simulink model "SixCellImplementation"  (R2021b)
settings: Solver=VariableStepAuto  StartTime=0.0  StopTime=500  RelTol=1e-3
libraries: spsVoltageMeasurementLib x8, spsDiodeLib x6, spsSeriesRLCBranchLib x6, spsLinearTransformerLib x3, spsGroundLib x1, spsMosfetLib x1, spspowerguiLib x1
settings Model: Creator=HP  LastModifiedBy=rajra
settings SolverCC: ZeroCrossAlgorithm=Adaptive  AlgebraicLoopSolver=TrustRegion
settings DebuggingCC: IgnoredZcDiagnostic=none  SFMachineParentedDataDiag=warning

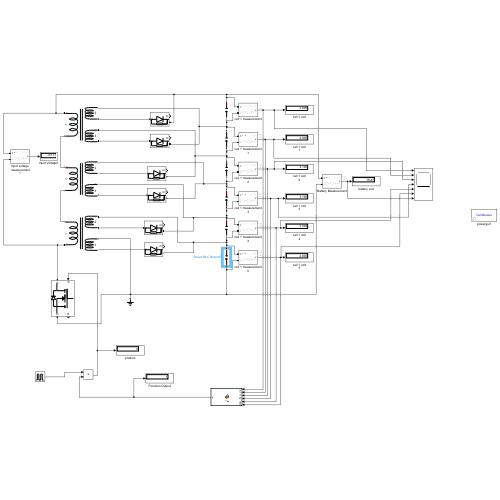
[thumbnail: Simulink's stored preview of the top-level diagram]
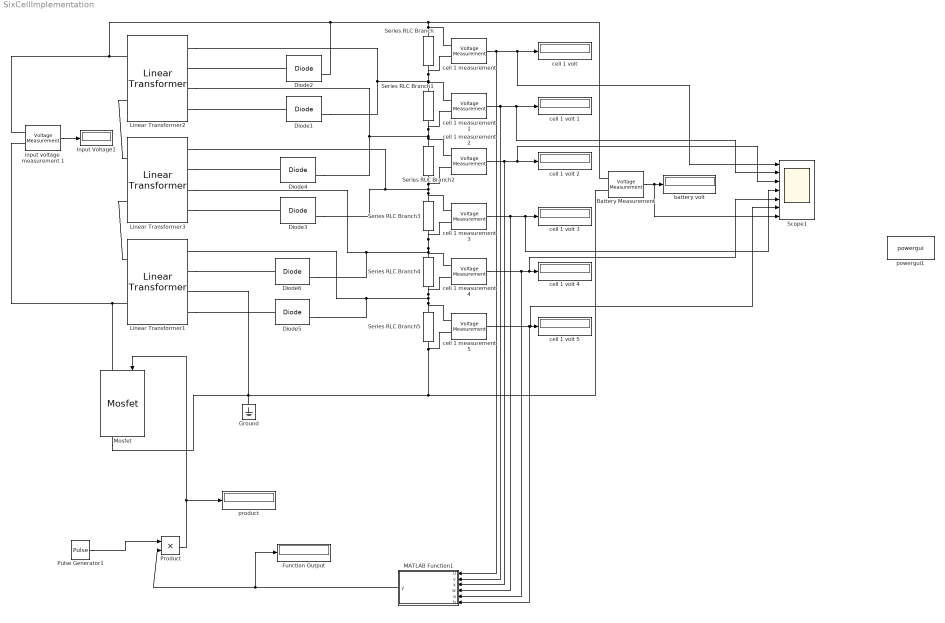
== system SixCellImplementation ==
  "Battery Measurement " : spsVoltageMeasurementLib/Voltage Measurement  PhasorSimulation=off  OutputType=Complex  PSBequivalent=0
  Diode{1..6} (6 alike) : spsDiodeLib/Diode  Ron=0.001  Lon=0  Vf=0.8  IC=0  UseSnubber=0  Rs=500  Cs=250e-9  Measurements=on
  Function Output : Display
  Ground : spsGroundLib/Ground  LConnTagsString=a
  Input Voltage1 : Display
  Linear Transformer1 : spsLinearTransformerLib/Linear Transformer  UNITS=SI  NominalPower=[100 55000]  winding1=[10 0.02 45e-6]  winding2=[5 0.02 288e-6]  ThreeWindings=on  winding3=[5 0.02 288e-6]  RmLm=[1.0805e+06 2866]  Measurements=None  DataType=on
  Linear Transformer2 : spsLinearTransformerLib/Linear Transformer  UNITS=SI  NominalPower=[100 55000]  winding1=[10 0.02 45e-6]  winding2=[5 0.02 288e-6]  ThreeWindings=on  winding3=[5 0.02 288e-6]  RmLm=[1.0805e+06 2866]  Measurements=None  DataType=on
  Linear Transformer3 : spsLinearTransformerLib/Linear Transformer  UNITS=SI  NominalPower=[100 55000]  winding1=[10 0.02 45e-6]  winding2=[5 0.02 288e-6]  ThreeWindings=on  winding3=[5 0.02 288e-6]  RmLm=[1.0805e+06 2866]  Measurements=None  DataType=on
  MATLAB Function1 : MATLAB Function  TreatAsAtomicUnit=on
  Mosfet : spsMosfetLib/Mosfet  Ron=1.5  Lon=0  Rd=2  Vfd=0  IC=0  Rs=1500  Cs=288e-7  Measurements=on
  Product : Product
  Pulse Generator1 : DiscretePulseGenerator  PulseType=Time based  Period=10  PulseWidth=50
  Scope1 : Scope  NumInputPorts=7
  Series RLC Branch : spsSeriesRLCBranchLib/Series RLC Branch  LConnTagsString=__new0  RConnTagsString=__new0  BranchType=C  Resistance=1  Inductance=1e-3  SetiL0=off  InitialCurrent=0  Capacitance=5  Setx0=on  InitialVoltage=3  Measurements=None
  Series RLC Branch1 : spsSeriesRLCBranchLib/Series RLC Branch  LConnTagsString=__new0  RConnTagsString=__new0  BranchType=C  Resistance=1  Inductance=1e-3  SetiL0=off  InitialCurrent=0  Capacitance=5  Setx0=on  InitialVoltage=3.0  Measurements=None
  Series RLC Branch2 : spsSeriesRLCBranchLib/Series RLC Branch  LConnTagsString=__new0  RConnTagsString=__new0  BranchType=C  Resistance=1  Inductance=1e-3  SetiL0=off  InitialCurrent=0  Capacitance=5  Setx0=on  InitialVoltage=3.2  Measurements=None
  Series RLC Branch3 : spsSeriesRLCBranchLib/Series RLC Branch  LConnTagsString=__new0  RConnTagsString=__new0  BranchType=C  Resistance=1  Inductance=1e-3  SetiL0=off  InitialCurrent=0  Capacitance=5  Setx0=on  InitialVoltage=3.2  Measurements=None
  Series RLC Branch4 : spsSeriesRLCBranchLib/Series RLC Branch  LConnTagsString=__new0  RConnTagsString=__new0  BranchType=C  Resistance=1  Inductance=1e-3  SetiL0=off  InitialCurrent=0  Capacitance=5  Setx0=on  InitialVoltage=3.1  Measurements=None
  Series RLC Branch5 : spsSeriesRLCBranchLib/Series RLC Branch  LConnTagsString=__new0  RConnTagsString=__new0  BranchType=C  Resistance=1  Inductance=1e-3  SetiL0=off  InitialCurrent=0  Capacitance=5  Setx0=on  InitialVoltage=3  Measurements=None
  "battery volt " : Display
  cell 1 measurement {,1..5} (6 alike) : spsVoltageMeasurementLib/Voltage Measurement  PhasorSimulation=off  OutputType=Complex  PSBequivalent=0
  cell 1 volt {,1..5} (6 alike) : Display
  input voltage measurement 1 : spsVoltageMeasurementLib/Voltage Measurement  PhasorSimulation=off  OutputType=Complex  PSBequivalent=0
  powergui1 : spspowerguiLib/powergui  Priority=1  SimulationMode=Continuous  SampleTime=50e-6  frequency=60  Iterations=50  frequencyindice=0  Pbase=100e6  ErrMax=1e-4  UnitsV=kV  UnitsW=MW  buscounter=0  FunctionMessages=off  echomessages=off  EnableUseOfTLC=off  CurrentSourceSwitches=off  DisableSnubberDevices=off  DisableRonSwitches=off  DisableVfSwitches=off  DisplayEquations=off  AutomaticDiscreteSolvers=off  SolverType=Tustin/Backward Euler (TBE)  Interpol=off  ExternalGateDelay=off  methode=off  Ts=100  x0status=blocks  SPID=on  SwTol=0  HookPort=off  NonlinearTolerance=1e-4  nMaxIteration=100  ContinueOnMaxIteration=off  RestoreLinks=warning  ResistiveCurrentMeasurement=off  Frange=[0:2:500]  Ylog=off  Xlog=on  ShowGrid=off  save=off  variable=ZData  structure=0  ZoomFFT=off  StartTime=0.0  cycles=1  DisplayStyle=1  fundamental=60  FreqAxis=off  MaxFrequency=1000  frequencyindicesteady=1  RmsSteady=1  display=off
  "product " : Display
  wires:
  input voltage measurement 1/1 -> Input Voltage1/1
  Pulse Generator1/1 -> Product/1
  MATLAB Function1/1(y) -> Function Output/1, Product/2
  Product/1 -> Mosfet/1, "product "/1
  "cell 1 measurement "/1 -> MATLAB Function1/1(u), Scope1/1, "cell 1 volt "/1
  cell 1 measurement 1/1 -> MATLAB Function1/2(v), Scope1/2, cell 1 volt 1/1
  cell 1 measurement 2/1 -> MATLAB Function1/3(x), Scope1/3, cell 1 volt 2/1
  cell 1 measurement 3/1 -> MATLAB Function1/4(w), Scope1/4, cell 1 volt 3/1
  cell 1 measurement 4/1 -> MATLAB Function1/5(a), Scope1/5, cell 1 volt 4/1
  cell 1 measurement 5/1 -> MATLAB Function1/6(b), Scope1/6, cell 1 volt 5/1
  "Battery Measurement "/1 -> Scope1/7, "battery volt "/1
  connections:
  Linear Transformer2/LConn2 -- Linear Transformer3/LConn1
  Linear Transformer3/LConn2 -- Linear Transformer1/LConn1
  Linear Transformer2/RConn2 -- Diode2/LConn1
  input voltage measurement 1/LConn1 -- "Battery Measurement "/LConn1 -- "cell 1 measurement "/LConn1 -- Series RLC Branch/LConn1 -- Diode2/RConn1 -- Linear Transformer2/LConn1
  Linear Transformer2/RConn4 -- Diode1/LConn1
  Series RLC Branch/RConn1 -- "cell 1 measurement "/LConn2 -- Linear Transformer2/RConn1 -- Diode1/RConn1 -- cell 1 measurement 1/LConn1 -- Series RLC Branch1/LConn1
  Series RLC Branch2/RConn1 -- cell 1 measurement 2/LConn2 -- Diode3/RConn1 -- Linear Transformer3/RConn1 -- cell 1 measurement 3/LConn1 -- Series RLC Branch3/LConn1
  Linear Transformer3/RConn4 -- Diode3/LConn1
  Linear Transformer3/RConn2 -- Diode4/LConn1
  Series RLC Branch1/RConn1 -- cell 1 measurement 1/LConn2 -- Linear Transformer2/RConn3 -- Diode4/RConn1 -- cell 1 measurement 2/LConn1 -- Series RLC Branch2/LConn1
  Series RLC Branch4/RConn1 -- cell 1 measurement 4/LConn2 -- Linear Transformer1/RConn1 -- Diode5/RConn1 -- cell 1 measurement 5/LConn1 -- Series RLC Branch5/LConn1
  Series RLC Branch3/RConn1 -- cell 1 measurement 3/LConn2 -- cell 1 measurement 4/LConn1 -- Linear Transformer3/RConn3 -- Diode6/RConn1 -- Series RLC Branch4/LConn1
  Linear Transformer1/RConn4 -- Diode5/LConn1
  Linear Transformer1/RConn2 -- Diode6/LConn1
  Linear Transformer1/LConn2 -- input voltage measurement 1/LConn2 -- Mosfet/LConn1
  Linear Transformer1/RConn3 -- "Battery Measurement "/LConn2 -- cell 1 measurement 5/LConn2 -- Series RLC Branch5/RConn1 -- Ground/LConn1 -- Mosfet/RConn1

== matlab function SixCellImplementation/MATLAB Function1 ==
  data: u input; y output; v input; x input; w input; a input; b input
function y = fcn(u,v,x,w,a,b)
if(u <= v && u >= v &&  v<= w && v>= w && v <= x && v >= x && v <= a && v >= a && v <= b && v >= b)
    y = 0;
else 
    y = 1;
end
